simulink model "izaje_carro_test"  (R2019a)
settings: Solver=VariableStepAuto  StartTime=0.0  StopTime=10.0  RelTol=1e-3
libraries: simulink x1
settings Model: Creator=Facundo  LastModifiedBy=Facundo

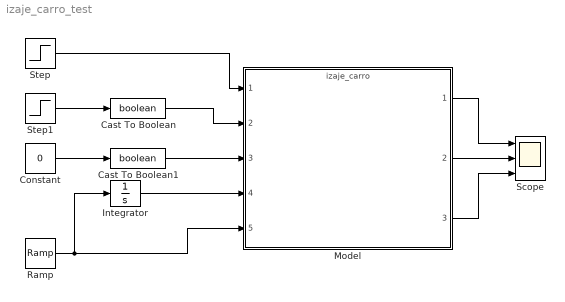
== system izaje_carro_test ==
  Cast To Boolean : DataTypeConversion  OutDataTypeStr=boolean
  Cast To Boolean1 : DataTypeConversion  OutDataTypeStr=boolean
  Constant : Constant  Value=0
  Integrator : Integrator
  Model : ModelReference  ModelNameDialog=izaje_carro.slx  SimulationMode=Normal  ShowModelTerminatePort=on  ModelReferenceVersion=1.37
  Ramp : simulink/Sources/Ramp  slope=1  start=0.5  InitialOutput=0
  Scope : Scope  NumInputPorts=3
  Step : Step  Time=0.5  SampleTime=0
  Step1 : Step  Time=7  SampleTime=0
  wires:
  Step/1 -> Model/1
  Step1/1 -> Cast To Boolean/1
  Constant/1 -> Cast To Boolean1/1
  Ramp/1 -> Integrator/1, Model/5
  Integrator/1 -> Model/4
  Model/1 -> Scope/1
  Model/2 -> Scope/2
  Model/3 -> Scope/3
  Cast To Boolean/1 -> Model/2
  Cast To Boolean1/1 -> Model/3
